simulink model "qpsk"  (R2016a)
settings: Solver=FixedStepDiscrete  SolverMode=SingleTasking  StartTime=0.0  StopTime=(12+49)*8  RelTol=1e-3
undefined symbols (not defined in the file or in its folder): rcosine
libraries: dspstat3 x1
settings Model: Creator=coltmt  LastModifiedBy=coltmt
settings DataIOCC: LimitDataPoints=on
settings DebuggingCC: AllowSymbolicDim=off
settings ModelReferenceCC: PropagateSignalLabelsOutOfModel=off
settings GRTTargetCC: GeneratePreprocessorConditionals=Use local settings

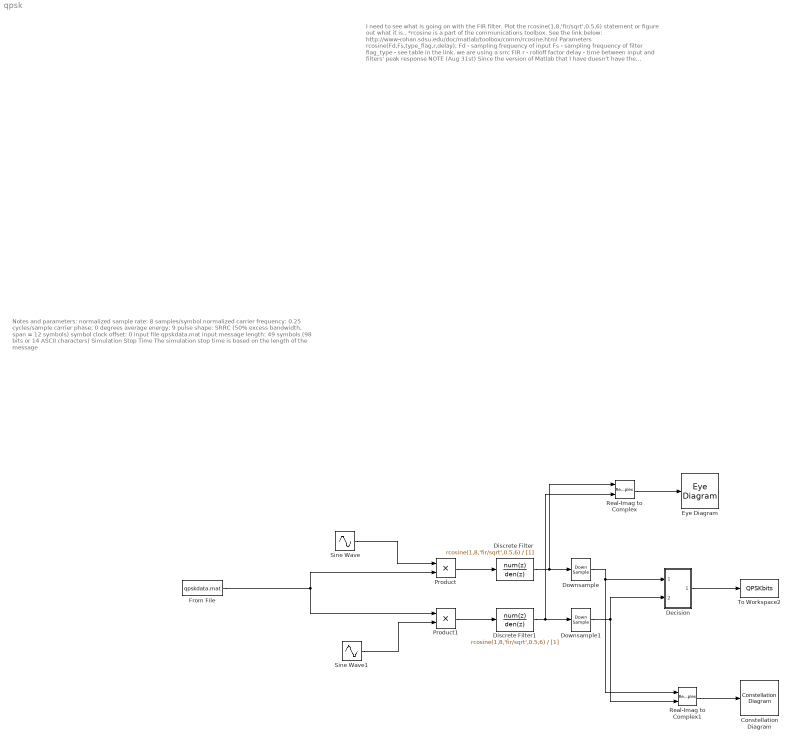
== system qpsk ==
  note: I need to see what is going on with the FIR filter. Plot
      | the rcosine(1,8,'fir/sqrt',0.5,6) statement or figure out what it is..
      |
      | *rcosine is a part of the communications toolbox. See the link below:
      | http://www-rohan.sdsu.edu/doc/matlab/toolbox/comm/rcosine.html
      |
      | Parameters rcosine(Fd,Fs,type_flag,r,delay);
      | Fd - sampling frequency of input
      | Fs - sampling frequency of filter
      | flag_type - see table in the link. we are using a srrc FIR
      | r - rolloff factor
      | delay - time between input and filters' peak response
      |
      | NOTE (Aug 31st)
      | Since the version of Matlab that I have duesn't have the communications toolbox I decided to use a different filter. We will see how it works:
      |
      | rcosdesign(beta,span,sps,shape)
      | beta - rolloff factor
      | span - input sample rate?
      | sps - filter sample rate?
      | shape - we will use 'sqrt'
      |
      | rcosdesign(0.5,1,8,'sqrt')
  note: Notes and parameters:
      | normalized sample rate: 8 samples/symbol
      | normalized carrier frequency: 0.25 cycles/sample
      | carrier phase: 0 degrees
      | average energy: 9
      | pulse shape: SRRC (50% excess bandwidth, span = 12 symbols)
      | symbol clock offset: 0
      | input file qpskdata.mat
      | input message length: 49 symbols (98 bits or 14 ASCII characters)
      |
      | Simulation Stop Time
      | The simulation stop time is based on the length of the message
  Constellation Diagram : ConstellationDiagram
  "Decision " : Subsystem
  Discrete Filter : DiscreteFilter  Numerator=rcosine(1,8,'fir/sqrt',0.5,6)  Denominator=[1]
  Discrete Filter1 : DiscreteFilter  Numerator=rcosine(1,8,'fir/sqrt',0.5,6)  Denominator=[1]
  Downsample : DownSample  N=8  InputProcessing=Inherited (this choice will be removed - see release notes)  RateOptions=Allow multirate processing
  Downsample1 : DownSample  N=8  InputProcessing=Inherited (this choice will be removed - see release notes)  RateOptions=Allow multirate processing
  Eye Diagram : EyeDiagram
  From File : FromFile  FileName=qpskdata.mat  SampleTime=1
  Product : Product
  Product1 : Product
  Real-Imag to Complex : RealImagToComplex
  Real-Imag to Complex1 : RealImagToComplex
  Sine Wave : Sin  Amplitude=sqrt(2)  Frequency=2*pi/4  Phase=pi/2  SampleTime=1
  Sine Wave1 : Sin  Amplitude=-sqrt(2)  Frequency=2*pi/4  SampleTime=1
  To Workspace2 : ToWorkspace  VariableName=QPSKbits  SampleTime=-1
      settings: Save2DSignal=2-D array (concatenate along first dimension)
  wires:
  Sine Wave1/1 -> Product1/2
  Sine Wave/1 -> Product/1
  From File/1 -> Product1/1, Product/2
  Product1/1 -> Discrete Filter1/1
  Product/1 -> Discrete Filter/1
  Discrete Filter/1 -> Real-Imag to Complex/1, Downsample/1
  Discrete Filter1/1 -> Real-Imag to Complex/2, Downsample1/1
  Downsample/1 -> "Decision "/1(In1), Real-Imag to Complex1/1
  Downsample1/1 -> "Decision "/2(In2), Real-Imag to Complex1/2
  Real-Imag to Complex/1 -> Eye Diagram/1
  Real-Imag to Complex1/1 -> Constellation Diagram/1
  "Decision "/1(Out1) -> To Workspace2/1

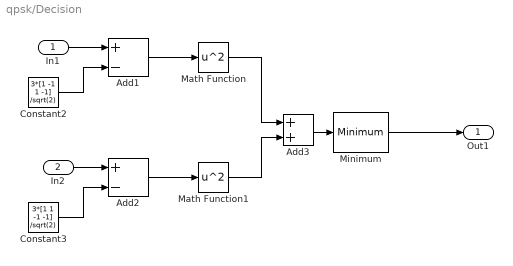
== system qpsk/Decision  ==
  In1 : Inport
  In2 : Inport  Port=2
  Add1 : Sum  Inputs=+-
  Add2 : Sum  Inputs=+-
  Add3 : Sum
  Constant2 : Constant  Value=3*[1 -1 1 -1] /sqrt(2)
  Constant3 : Constant  Value=3*[1 1 -1 -1] /sqrt(2)
  Math Function : Math  Operator=square  SaturateOnIntegerOverflow=on
  Math Function1 : Math  Operator=square  SaturateOnIntegerOverflow=on
  Minimum : dspstat3/Minimum  fcn=Index  reset=None  InputProcessing=Columns as channels (frame based)  indexBase=Zero  operateOver=Each column  Dimension=1  operation=minimum  roiEnable=off  roiType=Rectangles  roiPortion=Entire ROI  roiOutput=Individual statistics for each ROI  roiFlag=off  roundingMode=Floor  overflowMode=off
  Out1 : Outport
  wires:
  Math Function/1 -> Add3/1
  Math Function1/1 -> Add3/2
  Add3/1 -> Minimum/1
  Minimum/1 -> Out1/1
  Add1/1 -> Math Function/1
  Add2/1 -> Math Function1/1
  Constant3/1 -> Add2/2
  Constant2/1 -> Add1/2
  In1/1 -> Add1/1
  In2/1 -> Add2/1
